simulink model "Simul_LQR"  (R2020b)
settings: Solver=VariableStepAuto  StartTime=0.0  StopTime=40  RelTol=1e-3
values from neighbouring files (symbols this model uses):
  h = 0.01    [Unity3Dsimulacion.m]
undefined symbols (not defined in the file or in its folder): SetPoint, Ubar, X0, Xbar
libraries: cstblocks x1
settings Model: PauseTimes=0  Creator=Eduard  LastModifiedBy=Eduard

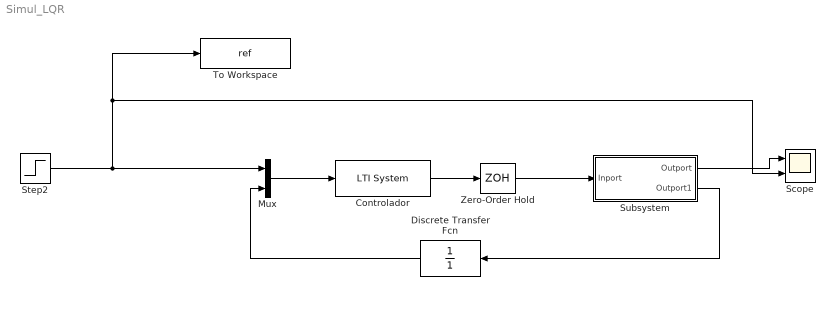
== system Simul_LQR ==
  Controlador : cstblocks/LTI System  sys=rL  IC=[]
  Discrete Transfer Fcn : DiscreteTransferFcn  Denominator=[1]  SampleTime=h
  Mux : Mux  Inputs=2
  Scope : Scope  NumInputPorts=2
  Step2 : Step  Time=0  After=SetPoint  SampleTime=0
  Subsystem : Subsystem
  To Workspace : ToWorkspace  VariableName=ref  SaveFormat=Structure With Time  SampleTime=-1
  Zero-Order Hold : ZeroOrderHold  SampleTime=h
  wires:
  Controlador/1 -> Zero-Order Hold/1
  Mux/1 -> Controlador/1
  Step2/1 -> Mux/1, To Workspace/1, Scope/2
  Subsystem/1(Outport) -> Scope/1
  Zero-Order Hold/1 -> Subsystem/1(Inport)
  Subsystem/2(Outport1) -> Discrete Transfer Fcn/1
  Discrete Transfer Fcn/1 -> Mux/2

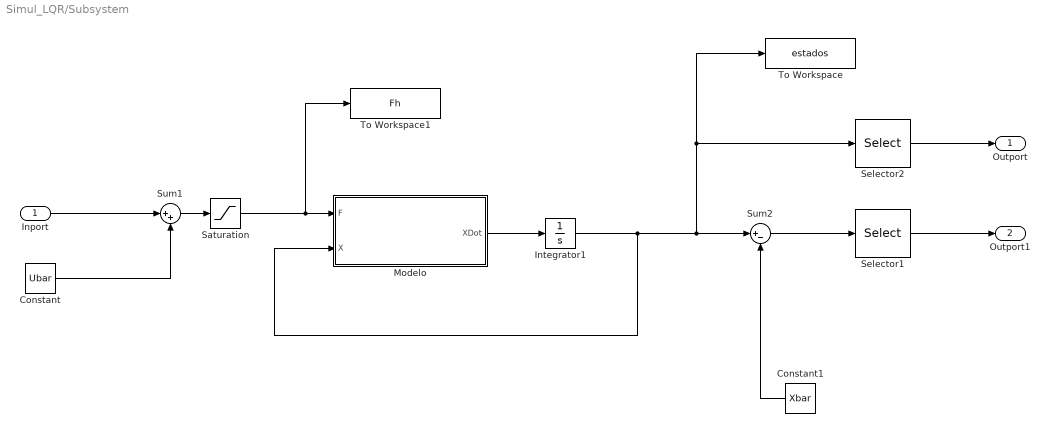
== system Simul_LQR/Subsystem ==
  Inport : Inport
  Constant : Constant  Value=Ubar
  Constant1 : Constant  Value=Xbar
  Integrator1 : Integrator  InitialCondition=X0
  Modelo : MATLAB Function  TreatAsAtomicUnit=on
  Saturation : Saturate  UpperLimit=0.25  LowerLimit=0
  Selector1 : Selector  InputPortWidth=6  IndexOptions=Index vector (dialog)  Indices=[3]  OutputSizes=1
  Selector2 : Selector  InputPortWidth=6  IndexOptions=Index vector (dialog)  Indices=[3]  OutputSizes=1
  Sum1 : Sum  Inputs=|++
  Sum2 : Sum  Inputs=|+-
  To Workspace : ToWorkspace  VariableName=estados  SaveFormat=Structure With Time  SampleTime=-1
  To Workspace1 : ToWorkspace  VariableName=Fh  SaveFormat=Structure With Time  SampleTime=h
  Outport : Outport
  Outport1 : Outport  Port=2
  wires:
  Constant/1 -> Sum1/2
  Inport/1 -> Sum1/1
  Constant1/1 -> Sum2/2
  Sum2/1 -> Selector1/1
  Selector2/1 -> Outport/1
  Selector1/1 -> Outport1/1
  Modelo/1(XDot) -> Integrator1/1
  Integrator1/1 -> Modelo/2(X), To Workspace/1, Selector2/1, Sum2/1
  Sum1/1 -> Saturation/1
  Saturation/1 -> To Workspace1/1, Modelo/1(F)

== matlab function Simul_LQR/Subsystem/Modelo ==
  data: F input; XDot output; X input
function XDot  = modelo_nolineal(F,X)
% Constantes del modelo
pc  = 1000;  % kg. m^-3 1000
ph  = 1000;
Vc  = 0.2;    % m^3
Vh  = 0.2;    % m^3
k   = 2*10^5; % J.°C^-1.min
Cc  = 4180;
Ch  = 4180;
Fc  = 0.05;   % m^3.min^-3 0.05
%Fh  = 0.11;   % m^3.min^-1 0.11
Tco = 20;     % °C 20
Tho = 90;     % °C. 90

% Estados
[Tc1, Tc2, Tc3, Th1, Th2, Th3]= deal(X(1),X(2),X(3),X(4),X(5),X(6));

% Derivadas de los estados
Tc1p = ( pc*Fc*Cc*(Tco-Tc1)  + k*(Th3-Tc1)) / (pc*Vc*Cc);
Tc2p = ( pc*Fc*Cc*(Tc1-Tc2)  + k*(Th2-Tc2)) / (pc*Vc*Cc);
Tc3p = ( pc*Fc*Cc*(Tc2-Tc3)  + k*(Th1-Tc3)) / (pc*Vc*Cc);

Th1p = ( ph*F*Ch*(Tho-Th1)  + k*(Tc3-Th1)) / (ph*Vh*Ch);
Th2p = ( ph*F*Ch*(Th1-Th2)  + k*(Tc2-Th2)) / (ph*Vh*Ch);
Th3p = ( ph*F*Ch*(Th2-Th3)  + k*(Tc1-Th3)) / (ph*Vh*Ch);


%% Modelo en espacio de estados
XDot                = [Tc1p; Tc2p; Tc3p; Th1p; Th2p; Th3p];
end
